simulink model "SIMQGC"  (R2017a)
settings: Solver=VariableStepAuto  StartTime=0.0  StopTime=1000  RelTol=1e-3
model workspace: external: MAT-File (data not in the file)
values from neighbouring files (symbols this model uses):
  aDe =     [MY3.mat]
  aDyn =     [MY3.mat]
  aLat =     [MY3.mat]
  aLon =     [MY3.mat]
  H = HGround + geo.Zgear + GearData.R - MCdata.mass*9.8/4/GearData.Sp    [my3_acdata.m]
  HGround = 500    [my3_acdata.m]
  phi_max = 20    [my3_acdata.m]
  phi_min = -20    [my3_acdata.m]
  psi_max = 30    [my3_acdata.m]
  psi_min = -30    [my3_acdata.m]
  theta_max = 20    [my3_acdata.m]
  theta_min = -20    [my3_acdata.m]
  Xmax = 0.01    [my3_acdata.m]
  Xmin = 0    [my3_acdata.m]
  Ymax = 0.01    [my3_acdata.m]
  Ymin = 0    [my3_acdata.m]
  Zmax = 0.01    [my3_acdata.m]
  Zmin = 0    [my3_acdata.m]
undefined symbols (not defined in the file or in its folder): Earth, geo, ini, magnitude, Motor, Newton, Prop, Raphson, Standard_Devices, UDP_Protocol, WGS84
undefined symbols (not defined in the file): GearData, LProp, RProp
libraries: simulink_extras x12, dspnetwork x8, aerolibobsolete x6, sharedutil x6, simulink x4, aerolibfltsims x3, aerolibasang x2, aerolibatmos2 x1, aerolibbdyn x1, aerolibtransform2 x1, aerolibanimutils x1, sldrtlib x1
(part 2 of 3)

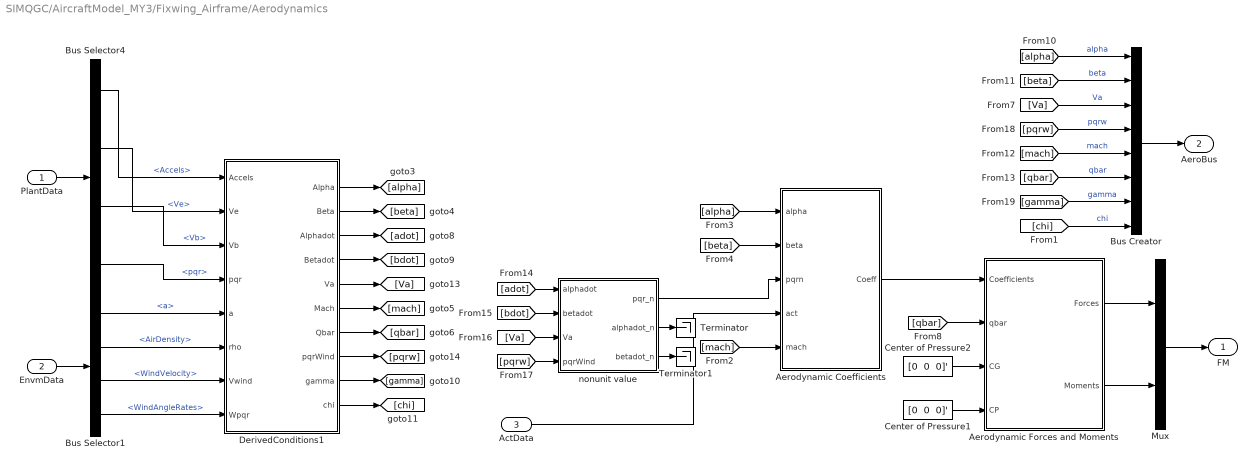
== system SIMQGC/AircraftModel_MY3/Fixwing_Airframe/Aerodynamics ==
  PlantData : Inport
  EnvmData : Inport  Port=2
  ActData : Inport  Port=3
  Aerodynamic Coefficients : Subsystem  AncestorBlock=asbhl20vehicle/Vehicle/Aerodynamic/Aerodynamic Coefficients
  Aerodynamic Forces and Moments : Subsystem  mask(Aerodynamic Forces and Moments){S=geo.Sw, b=geo.b, cbar=geo.MAC}
      mask prompts: S "Reference area:"; b "Reference span:"; cbar "Reference length:"
      mask help: Compute the aerodynamic forces and moments applied at the center of gravity using the aerodynamic coefficients, dynamic pressure, center of gravity and center of pressure.
      mask Help: web(asbhelp);
      mask Display:
      | port_label('input',1,'Coefficients','texmode','on');
      | port_label('input',2,'q_{bar}','texmode','on');
      | port_label('input',3,'CG','texmode','on');
      | port_label('input',4,'CP','texmode','on');
      | port_label('output',1,'F_{aero}','texmode','on');
      | port_label('output',2,'M_{aero}','texmode','on');
  Bus Creator : BusCreator  Inputs=8
  Bus Selector1 : BusSelector  OutputSignals=a,AirDensity,WindVelocity,WindAngleRates
  Bus Selector4 : BusSelector  OutputSignals=Accels,Ve,Vb,pqr
  Center of Pressure1 : Constant  Value="[0  0  0]'"  SampleTime=0
  Center of Pressure2 : Constant  Value="[0  0  0]'"  SampleTime=0
  DerivedConditions1 : Subsystem
  Mux : Mux  Inputs=2
  Terminator : Terminator
  Terminator1 : Terminator
  nonunit value : Subsystem
  FM : Outport  PortDimensions=6
  AeroBus : Outport  Port=2
  wires:
  Aerodynamic Forces and Moments/1(Forces) -> Mux/1
  PlantData/1 -> Bus Selector4/1
  EnvmData/1 -> Bus Selector1/1
  Bus Creator/1 -> AeroBus/1
  [qbar] -> Aerodynamic Forces and Moments/2(qbar)
  Bus Selector4/1 -> DerivedConditions1/1(Accels)  "<Accels>"
  Bus Selector4/2 -> DerivedConditions1/2(Ve)  "<Ve>"
  Bus Selector4/3 -> DerivedConditions1/3(Vb)  "<Vb>"
  Bus Selector4/4 -> DerivedConditions1/4(pqr)  "<pqr>"
  Bus Selector1/1 -> DerivedConditions1/5(a)  "<a>"
  Bus Selector1/2 -> DerivedConditions1/6(rho)  "<AirDensity>"
  Bus Selector1/3 -> DerivedConditions1/7(Vwind)  "<WindVelocity>"
  Bus Selector1/4 -> DerivedConditions1/8(Wpqr)  "<WindAngleRates>"
  DerivedConditions1/1(Alpha) -> [alpha]
  DerivedConditions1/2(Beta) -> [beta]
  DerivedConditions1/5(Va) -> [Va]
  DerivedConditions1/6(Mach) -> [mach]
  DerivedConditions1/7(Qbar) -> [qbar]
  DerivedConditions1/8(pqrWind) -> [pqrw]
  DerivedConditions1/9(gamma) -> [gamma]
  DerivedConditions1/10(chi) -> [chi]
  [alpha] -> Bus Creator/1  "alpha"
  [beta] -> Bus Creator/2  "beta"
  [Va] -> Bus Creator/3  "Va"
  [pqrw] -> Bus Creator/4  "pqrw"
  [mach] -> Bus Creator/5  "mach"
  [qbar] -> Bus Creator/6  "qbar"
  [gamma] -> Bus Creator/7  "gamma"
  Aerodynamic Forces and Moments/2(Moments) -> Mux/2
  Mux/1 -> FM/1
  DerivedConditions1/3(Alphadot) -> [adot]
  DerivedConditions1/4(Betadot) -> [bdot]
  [adot] -> nonunit value/1(alphadot)
  [bdot] -> nonunit value/2(betadot)
  [Va] -> nonunit value/3(Va)
  [pqrw] -> nonunit value/4(pqrWind)
  [alpha] -> Aerodynamic Coefficients/1(alpha)
  [beta] -> Aerodynamic Coefficients/2(beta)
  nonunit value/1(pqr_n) -> Aerodynamic Coefficients/3(pqrn)
  nonunit value/2(alphadot_n) -> Terminator/1
  nonunit value/3(betadot_n) -> Terminator1/1
  Center of Pressure2/1 -> Aerodynamic Forces and Moments/3(CG)
  Center of Pressure1/1 -> Aerodynamic Forces and Moments/4(CP)
  ActData/1 -> Aerodynamic Coefficients/4(act)
  [chi] -> Bus Creator/8  "chi"
  [mach] -> Aerodynamic Coefficients/5(mach)
  Aerodynamic Coefficients/1(Coeff) -> Aerodynamic Forces and Moments/1(Coefficients)

== system SIMQGC/AircraftModel_MY3/Fixwing_Airframe/Gravity ==
  PlantData : Inport
  Bus Selector1 : BusSelector  OutputSignals=gb
  Constant1 : Constant  Value=ini.mass
  Constant3 : Constant  Value=[0 0 0]'
  Constant4 : Constant  Value=geo.Xcg
  Constant5 : Constant  Value=0
  Constant6 : Constant  Value=0
  Mux1 : Mux  Inputs=2
  Mux2 : Mux  Inputs=3
  Product : Product  RndMeth=Zero
  FM : Outport  PortDimensions=6
  mass : Outport  Port=2
  CG : Outport  Port=3
  wires:
  PlantData/1 -> Bus Selector1/1
  Constant3/1 -> Mux1/2
  Mux1/1 -> FM/1
  Bus Selector1/1 -> Product/1  "<gb>"
  Product/1 -> Mux1/1
  Constant1/1 -> Product/2, mass/1
  Mux2/1 -> CG/1
  Constant4/1 -> Mux2/1
  Constant5/1 -> Mux2/2
  Constant6/1 -> Mux2/3

== system SIMQGC/AircraftModel_MY3/Fixwing_Airframe/GroundForces ==
  PlantData : Inport
  Bus Creator : BusCreator  Inputs=4
  Constant : Constant  Value=HGround
  LF_Gear : Subsystem  AncestorBlock=|  TreatAsAtomicUnit=on  mask(simple aircraft undercarriage){loc=GearData.PLF, Rw=GearData.R, Ks=GearData.Sp, Cs=GearData.Damp, Rcs=GearData.CompMax, muroll=GearData.muRoll, A=GearData.muA, B=GearData.muB}
      | asbhl20vehicle/Vehicle/LandingGear
      | GroundReaction/L Main Gear Geometry
      | Forces and Moments
      mask prompts: loc "Gear location"; Rw "Wheel radius"; Ks "Strut Spring rate"; Cs "Strut Damping rate"; Rcs "Strut compress range"; muroll "Tire roll friction coefficient"; A "Tire friction caculate experience formula parameter A"; B "Tire friction caculate experience formula parameter B"
      mask help:
      | the model descripes the basic mechanics model according to  geoometry
      | relationship. there are no brake device model, and no hydraulic model etc,
      | only the basic forces and moments caculation in the model.
      | it is designed to be appllied to small uav.
  LM_Gear : Subsystem  AncestorBlock=|  TreatAsAtomicUnit=on  mask(simple aircraft undercarriage){loc=GearData.PLM, Rw=GearData.R, Ks=GearData.Sp, Cs=GearData.Damp, Rcs=GearData.CompMax, muroll=GearData.muRoll, A=GearData.muA, B=GearData.muB}
      | asbhl20vehicle/Vehicle/LandingGear
      | GroundReaction/L Main Gear Geometry
      | Forces and Moments
      mask prompts: loc "Gear location"; Rw "Wheel radius"; Ks "Strut Spring rate"; Cs "Strut Damping rate"; Rcs "Strut compress range"; muroll "Tire roll friction coefficient"; A "Tire friction caculate experience formula parameter A"; B "Tire friction caculate experience formula parameter B"
      mask help:
      | the model descripes the basic mechanics model according to  geoometry
      | relationship. there are no brake device model, and no hydraulic model etc,
      | only the basic forces and moments caculation in the model.
      | it is designed to be appllied to small uav.
  LN_Gear : Subsystem  AncestorBlock=|  TreatAsAtomicUnit=on  mask(simple aircraft undercarriage){loc=GearData.PRM, Rw=GearData.R, Ks=GearData.Sp, Cs=GearData.Damp, Rcs=GearData.CompMax, muroll=GearData.muRoll, A=GearData.muA, B=GearData.muB}
      | asbhl20vehicle/Vehicle/LandingGear
      | GroundReaction/L Main Gear Geometry
      | Forces and Moments
      mask prompts: loc "Gear location"; Rw "Wheel radius"; Ks "Strut Spring rate"; Cs "Strut Damping rate"; Rcs "Strut compress range"; muroll "Tire roll friction coefficient"; A "Tire friction caculate experience formula parameter A"; B "Tire friction caculate experience formula parameter B"
      mask help:
      | the model descripes the basic mechanics model according to  geoometry
      | relationship. there are no brake device model, and no hydraulic model etc,
      | only the basic forces and moments caculation in the model.
      | it is designed to be appllied to small uav.
  RF_Gear : Subsystem  AncestorBlock=|  TreatAsAtomicUnit=on  mask(simple aircraft undercarriage){loc=GearData.PRF, Rw=GearData.R, Ks=GearData.Sp, Cs=GearData.Damp, Rcs=GearData.CompMax, muroll=GearData.muRoll, A=GearData.muA, B=GearData.muB}
      | asbhl20vehicle/Vehicle/LandingGear
      | GroundReaction/L Main Gear Geometry
      | Forces and Moments
      mask prompts: loc "Gear location"; Rw "Wheel radius"; Ks "Strut Spring rate"; Cs "Strut Damping rate"; Rcs "Strut compress range"; muroll "Tire roll friction coefficient"; A "Tire friction caculate experience formula parameter A"; B "Tire friction caculate experience formula parameter B"
      mask help:
      | the model descripes the basic mechanics model according to  geoometry
      | relationship. there are no brake device model, and no hydraulic model etc,
      | only the basic forces and moments caculation in the model.
      | it is designed to be appllied to small uav.
  Sum : Sum  Inputs=++++
  Terminator{,1..3} (4 alike) : Terminator
  FM : Outport
  WOW : Outport  Port=2
  wires:
  PlantData/1 -> RF_Gear/1(PlantData), LN_Gear/1(PlantData), LM_Gear/1(PlantData), LF_Gear/1(PlantData)
  Constant/1 -> RF_Gear/2(runway height), LN_Gear/2(runway height), LM_Gear/2(runway height), LF_Gear/2(runway height)
  LF_Gear/3(FM) -> Sum/1
  RF_Gear/3(FM) -> Sum/2
  LM_Gear/3(FM) -> Sum/3
  LN_Gear/3(FM) -> Sum/4
  Sum/1 -> FM/1
  LF_Gear/1(WOW) -> [LF]
  RF_Gear/1(WOW) -> [RF]
  LM_Gear/1(WOW) -> [LM]
  LN_Gear/1(WOW) -> [RM]
  [RF] -> Bus Creator/2  "RF"
  Bus Creator/1 -> WOW/1
  [LF] -> Bus Creator/1  "LF"
  [LM] -> Bus Creator/3  "LM"
  [RM] -> Bus Creator/4  "RM"
  LF_Gear/2(S) -> Terminator/1
  RF_Gear/2(S) -> Terminator1/1
  LM_Gear/2(S) -> Terminator2/1
  LN_Gear/2(S) -> Terminator3/1

== system SIMQGC/AircraftModel_MY3/Fixwing_Airframe/PlantBus ==
  Ve : Inport
  Xe : Inport  Port=2
  Euler : Inport  Port=3
  DCM : Inport  Port=4
  Vb : Inport  Port=5
  pqr : Inport  Port=6
  pqrdot : Inport  Port=7
  Accels : Inport  Port=8
  AeroBus : Inport  Port=9
  EnvmData : Inport  Port=10
  mass : Inport  Port=11
  CG : Inport  Port=12
  ACTData : Inport  Port=13
  WOW : Inport  Port=14
  5 : Selector  InputPortWidth=3  IndexOptions=Index vector (dialog)  Indices=3  OutputSizes=1
  Bus Selector1 : BusSelector  OutputSignals=alpha,beta,Va,pqrw,mach,qbar,gamma,chi
  Bus Selector4 : BusSelector  OutputSignals=hground,g,To,Po
  Gain : Gain  Gain=-1
  PlantBus : BusCreator  Inputs=26
  Subsystem : Subsystem
  Sum : Sum  Inputs=+-|
  "nb & gb " : Subsystem
  Data : Outport
  wires:
  Euler/1 -> Subsystem/1(Ein)
  PlantBus/1 -> Data/1  "PlantBus"
  AeroBus/1 -> Bus Selector1/1
  EnvmData/1 -> Bus Selector4/1
  Ve/1 -> PlantBus/1  "Ve"
  Xe/1 -> PlantBus/2, 5/1  "Xe"
  5/1 -> Gain/1
  Gain/1 -> PlantBus/3, Sum/1  "H"
  DCM/1 -> PlantBus/6, "nb & gb "/1(DCM)  "DCM"
  Bus Selector4/1 -> Sum/2  "<hground>"
  Accels/1 -> PlantBus/20, "nb & gb "/3(a)  "Accels"
  Bus Selector4/2 -> "nb & gb "/2(g)  "<g>"
  Sum/1 -> PlantBus/4  "Hag"
  Subsystem/1(E) -> PlantBus/5  "Euler"
  Vb/1 -> PlantBus/7  "Vb"
  pqr/1 -> PlantBus/8  "pqr"
  pqrdot/1 -> PlantBus/9  "pqrdot"
  "nb & gb "/1(nb) -> PlantBus/10  "nb"
  "nb & gb "/2(gb) -> PlantBus/11  "gb"
  Bus Selector1/1 -> PlantBus/12  "<alpha>"
  Bus Selector1/2 -> PlantBus/13  "<beta>"
  Bus Selector1/3 -> PlantBus/14  "<Va>"
  Bus Selector1/4 -> PlantBus/15  "<pqrw>"
  Bus Selector1/5 -> PlantBus/16  "<mach>"
  Bus Selector1/6 -> PlantBus/17  "<qbar>"
  Bus Selector1/7 -> PlantBus/18  "<gamma>"
  Bus Selector1/8 -> PlantBus/19  "<chi>"
  mass/1 -> PlantBus/21  "mass"
  CG/1 -> PlantBus/22  "CG"
  ACTData/1 -> PlantBus/23  "ACTData"
  WOW/1 -> PlantBus/24  "WOW"
  Bus Selector4/3 -> PlantBus/25  "<To>"
  Bus Selector4/4 -> PlantBus/26  "<Po>"

== system SIMQGC/AircraftModel_MY3/Fixwing_Airframe/Propulsion ==
  ActData : Inport
  PlantData : Inport  Port=2
  EnvData : Inport  Port=3
  ActData1 : InportShadow
  Bus Selector : BusSelector  OutputSignals=dtl
  Bus Selector1 : BusSelector  OutputSignals=Va
  Bus Selector2 : BusSelector  OutputSignals=AirDensity
  Bus Selector3 : BusSelector  OutputSignals=dtr
  Bus Selector4 : BusSelector  OutputSignals=pqr
  Gain : Gain  Gain=Prop.Y
  Left_MotorAndPropeller : Subsystem  mask{P=LProp.P, C=LProp.C}
      mask prompts: P "Assemble Position in Body Frame(m)"; C "Spin Direction(-1 for clockwise,1 for countted clockwise)"
      mask DialogControl DescTextVar Prompt: Motor and Propeller Model
  Right_MotorAndPropeller : Subsystem  mask{P=RProp.P, C=RProp.C}
      mask prompts: P "Assemble Position in Body Frame(m)"; C "Spin Direction(-1 for clockwise,1 for countted clockwise)"
      mask DialogControl DescTextVar Prompt: Motor and Propeller Model
  Selector : Selector  InputPortWidth=3  IndexOptions=Index vector (dialog)  Indices=[3]  OutputSizes=1
  Sum : Sum  Inputs=|++
  Sum1 : Sum  Inputs=|++
  Sum2 : Sum  Inputs=+-|
  FM : Outport  PortDimensions=6  InitialOutput=0
  wires:
  ActData/1 -> Bus Selector/1
  PlantData/1 -> Bus Selector4/1, Bus Selector1/1
  Bus Selector/1 -> Left_MotorAndPropeller/1(dt)  "<dtl>"
  Bus Selector1/1 -> Sum2/1, Sum1/1  "<Va>"
  EnvData/1 -> Bus Selector2/1
  Bus Selector2/1 -> Right_MotorAndPropeller/3(rho), Left_MotorAndPropeller/3(rho)  "<AirDensity>"
  ActData1/1 -> Bus Selector3/1
  Bus Selector3/1 -> Right_MotorAndPropeller/1(dt)  "<dtr>"
  Left_MotorAndPropeller/1(FM) -> Sum/1
  Right_MotorAndPropeller/1(FM) -> Sum/2
  Sum/1 -> FM/1
  Sum1/1 -> Left_MotorAndPropeller/2(V)
  Bus Selector4/1 -> Selector/1  "<pqr>"
  Selector/1 -> Gain/1
  Gain/1 -> Sum2/2, Sum1/2
  Sum2/1 -> Right_MotorAndPropeller/2(V)

== system SIMQGC/UDPReadFromQGC/Subsystem/joystick ==
  data : Inport
  Action Port : ActionPort  ActionType=case
  Demux : Demux  Outputs=8
  Mux : Mux  Inputs=3
  Terminator{,1..4} (5 alike) : Terminator
  joystick : Outport
  wires:
  data/1 -> Demux/1
  Demux/1 -> Mux/1
  Demux/2 -> Mux/2
  Demux/3 -> Mux/3
  Mux/1 -> joystick/1
  Demux/4 -> Terminator/1
  Demux/5 -> Terminator1/1
  Demux/6 -> Terminator2/1
  Demux/7 -> Terminator3/1
  Demux/8 -> Terminator4/1

== system SIMQGC/UDPReadFromQGC/Subsystem/throttle ==
  data : Inport
  Action Port : ActionPort  ActionType=case
  Demux : Demux  Outputs=8
  Mux : Mux  Inputs=2
  Terminator{,1..5} (6 alike) : Terminator
  throttle : Outport
  wires:
  data/1 -> Demux/1
  Demux/1 -> Mux/1
  Demux/2 -> Mux/2
  Demux/3 -> Terminator5/1
  Mux/1 -> throttle/1
  Demux/4 -> Terminator/1
  Demux/5 -> Terminator1/1
  Demux/6 -> Terminator2/1
  Demux/7 -> Terminator3/1
  Demux/8 -> Terminator4/1

== system SIMQGC/AircraftModel_MY3/Fixwing_Airframe/Aerodynamics/Aerodynamic Coefficients ==
  alpha : Inport
  beta : Inport  Port=2
  pqrn : Inport  Port=3
  act : Inport  Port=4
  mach : Inport  Port=5
  Basic Coefficients : Subsystem
  Body Rate Damping : Subsystem
  LY0 : Gain
  LY1 : Gain
  Mux1 : Mux  Inputs=2
  Selector : Selector  InputPortWidth=6  IndexOptions=Index vector (dialog)  Indices=[1 2 3]  OutputSizes=1
  Selector1 : Selector  InputPortWidth=6  IndexOptions=Index vector (dialog)  Indices=[4 5 6]  OutputSizes=1
  Sum : Sum  Inputs=3  SaturateOnIntegerOverflow=on  InputSameDT=on  OutDataTypeStr=Inherit: Same as first input
  actuator : Subsystem
  body axis forces : Subsystem
  Coeff : Outport  InitialOutput=0
  wires:
  alpha/1 -> body axis forces/1(alpha), Body Rate Damping/1(alpha), actuator/1(alpha), Basic Coefficients/1(alpha)
  beta/1 -> body axis forces/2(beta), Basic Coefficients/2(beta)
  pqrn/1 -> Body Rate Damping/2(pqrn)
  Body Rate Damping/1(coeff) -> Sum/2
  Basic Coefficients/1(coeff) -> Sum/1
  actuator/1(coeff) -> Sum/3
  act/1 -> actuator/2(act)
  mach/1 -> Basic Coefficients/3(mach)
  Selector1/1 -> LY1/1
  Mux1/1 -> Coeff/1
  Selector/1 -> LY0/1
  Sum/1 -> Selector1/1, Selector/1
  body axis forces/1(Cl_XYZ) -> Mux1/1
  LY0/1 -> body axis forces/3(Cl_LDY)
  LY1/1 -> Mux1/2

== system SIMQGC/AircraftModel_MY3/Fixwing_Airframe/Aerodynamics/Aerodynamic Forces and Moments ==
  Coefficients : Inport
  qbar : Inport  Port=2
  CG : Inport  Port=3
  CP : Inport  Port=4
  Demux1 : Demux  Outputs=[3,3]
  Moments about CG due to Forces : aerolibbdyn/Moments about CG  due to Forces
      settings: SourceProductName=Aerospace Blockset  SourceProductBaseCode=AE
  Product : Product  SaturateOnIntegerOverflow=on  InputSameDT=on  OutDataTypeStr=Inherit: Same as first input
  Product3 : Product  SaturateOnIntegerOverflow=on  InputSameDT=on  OutDataTypeStr=Inherit: Same as first input
  Sum1 : Sum  Inputs=++|  SaturateOnIntegerOverflow=on  InputSameDT=on  OutDataTypeStr=Inherit: Same as first input
  reference area : Gain  Gain=S  SaturateOnIntegerOverflow=on  OutDataTypeStr=Inherit: Same as input  ParamDataTypeStr=Inherit: Same as input
  reference length : Gain  Gain=[b cbar b]  SaturateOnIntegerOverflow=on  OutDataTypeStr=Inherit: Same as input  ParamDataTypeStr=Inherit: Same as input
  Forces : Outport
  Moments : Outport  Port=2
  wires:
  Moments about CG due to Forces/1 -> Sum1/1
  reference length/1 -> Product3/2
  Coefficients/1 -> Demux1/1
  Demux1/1 -> Product/2
  Demux1/2 -> Product3/1
  qbar/1 -> reference area/1
  reference area/1 -> reference length/1, Product/1
  Product/1 -> Forces/1, Moments about CG due to Forces/1
  Product3/1 -> Sum1/2
  Sum1/1 -> Moments/1
  CG/1 -> Moments about CG due to Forces/2
  CP/1 -> Moments about CG due to Forces/3

== system SIMQGC/AircraftModel_MY3/Fixwing_Airframe/Aerodynamics/DerivedConditions1 ==
  Accels : Inport
  Ve : Inport  Port=2
  Vb : Inport  Port=3
  pqr : Inport  Port=4
  a : Inport  Port=5
  rho : Inport  Port=6
  Vwind : Inport  Port=7
  Wpqr : Inport  Port=8
  Derivative : Derivative
  Derivative1 : Derivative
  Dynamic Pressure : aerolibasang/Dynamic Pressure
  "Incidence, Sideslip, & Airspeed" : Subsystem  AncestorBlock=aerolibasang/Incidence, Sideslip, & Airspeed  mask(Incidence,Sideslip,&Airspeed){}
      mask help: aeroblks:aeroblkasang:blockIncidenceSideslipAirspeedDesc
      mask init:
      | aeroicon('aeroblk');
      mask Help: eval('asbhelp(''incidence_sideslip_and_airspeed'')');
      mask Display:
      | port_label('input',1,'V_b','texmode','on');
      | port_label('output',1,'\alpha','texmode','on');
      | port_label('output',2,'\beta','texmode','on');
      | port_label('output',3,'V','texmode','on');
  Mach Number : aerolibasang/Mach Number
      settings: SourceProductName=Aerospace Blockset  SourceProductBaseCode=AE
  Saturation1 : Saturate  UpperLimit=40/57.3  LowerLimit=-40/57.3
  Sum1 : Sum  Inputs=++|  SaturateOnIntegerOverflow=on  InputSameDT=on  OutDataTypeStr=Inherit: Same as first input
  Sum2 : Sum  Inputs=|+-  SaturateOnIntegerOverflow=on  InputSameDT=on  OutDataTypeStr=Inherit: Same as first input
  Terminator : Terminator
  Terminator1 : Terminator
  Terminator2 : Terminator
  gamma chi & speed : Subsystem  AncestorBlock=cldesignlib/Aircraft Dynamics/gamma chi & speed  mask(flight path angle & speed){}
      mask help: Calculate the angles between the velocity vector and the ground under NED coordinate (Ve).
      mask Display:
      | port_label('input',1,'V_e','texmode','on');
      | port_label('output',1,'\gamma','texmode','on');
      | port_label('output',2,'\chi','texmode','on');
      | port_label('output',3,'V','texmode','on');
  pqr1 : InportShadow  Port=4
  Alpha : Outport
  Beta : Outport  Port=2
  Alphadot : Outport  Port=3
  Betadot : Outport  Port=4
  Va : Outport  Port=5
  Mach : Outport  Port=6
  Qbar : Outport  Port=7
  pqrWind : Outport  Port=8
  gamma : Outport  Port=9
  chi : Outport  Port=10
  wires:
  gamma chi & speed/2(chi) -> chi/1
  gamma chi & speed/1(gamma) -> gamma/1
  Ve/1 -> gamma chi & speed/1(Ve)
  Vwind/1 -> Sum2/2
  "Incidence, Sideslip, & Airspeed"/1(Alpha) -> Alpha/1, Derivative/1
  Sum1/1 -> pqrWind/1
  pqr/1 -> Sum1/1
  Wpqr/1 -> Sum1/2
  rho/1 -> Dynamic Pressure/2
  a/1 -> Mach Number/2
  Vb/1 -> Sum2/1
  Mach Number/1 -> Mach/1
  "Incidence, Sideslip, & Airspeed"/3(V) -> Va/1
  "Incidence, Sideslip, & Airspeed"/2(Beta) -> Saturation1/1
  Sum2/1 -> "Incidence, Sideslip, & Airspeed"/1(Vb), Dynamic Pressure/1, Mach Number/1
  Saturation1/1 -> Beta/1, Derivative1/1
  Derivative/1 -> Alphadot/1
  Derivative1/1 -> Betadot/1
  Dynamic Pressure/1 -> Qbar/1
  gamma chi & speed/3(V) -> Terminator2/1
  pqr1/1 -> Terminator/1
  Accels/1 -> Terminator1/1

== system SIMQGC/AircraftModel_MY3/Fixwing_Airframe/Aerodynamics/nonunit value ==
  alphadot : Inport
  betadot : Inport  Port=2
  Va : Inport  Port=3
  pqrWind : Inport  Port=4
  Demux2 : Demux  Outputs=3
  Gain : Gain  Gain=2  SaturateOnIntegerOverflow=on  OutDataTypeStr=Inherit: Same as input  ParamDataTypeStr=Inherit: Same as input
  Mux18 : Mux  Inputs=3
  Product{1..5} (5 alike) : Product  Inputs=/**  SaturateOnIntegerOverflow=on  OutDataTypeStr=Inherit: Same as first input
  Saturation : Saturate  UpperLimit=inf  LowerLimit=0.1
  b : Constant  Value=geo.b
  c : Constant  Value=geo.MAC
  pqr_n : Outport
  alphadot_n : Outport  Port=2
  betadot_n : Outport  Port=3
  wires:
  alphadot/1 -> Product3/3
  Product3/1 -> alphadot_n/1
  Saturation/1 -> Product2/1, Product3/1, Product5/1, Product4/1, Product1/1
  Product1/1 -> Mux18/1
  Mux18/1 -> pqr_n/1
  c/1 -> Product3/2, Product4/2
  Demux2/1 -> Product1/3
  Demux2/2 -> Product4/3
  Demux2/3 -> Product2/3
  b/1 -> Product1/2, Product2/2, Product5/2
  Gain/1 -> Saturation/1
  Product2/1 -> Mux18/3
  Product4/1 -> Mux18/2
  Va/1 -> Gain/1
  pqrWind/1 -> Demux2/1
  betadot/1 -> Product5/3
  Product5/1 -> betadot_n/1

== system SIMQGC/AircraftModel_MY3/Fixwing_Airframe/GroundForces/LF_Gear ==
  PlantData : Inport
  runway height : Inport  Port=2
  Bus Selector1 : BusSelector  OutputSignals=DCM,Xe,Vb,pqr,Euler
  Gain2 : Gain  Gain=-1
  GenerateGroundFM1 : Subsystem  TreatAsAtomicUnit=on
  detect ground contact : Subsystem
  gear location : Constant  Value=loc
  psi : Selector  InputPortWidth=3  IndexOptions=Index vector (dialog)  Indices=3  OutputSizes=1
  ze : Selector  InputPortWidth=3  IndexOptions=Index vector (dialog)  Indices=3  OutputSizes=1
  WOW : Outport
  S : Outport  Port=2
  FM : Outport  Port=3
  wires:
  GenerateGroundFM1/1(S) -> S/1
  Gain2/1 -> GenerateGroundFM1/1(zrw)
  gear location/1 -> GenerateGroundFM1/2(Xgb), detect ground contact/3(Xgb)
  psi/1 -> GenerateGroundFM1/7(psi)
  Bus Selector1/4 -> GenerateGroundFM1/6(pqr)  "<pqr>"
  Bus Selector1/3 -> GenerateGroundFM1/5(Vb)  "<Vb>"
  Bus Selector1/1 -> GenerateGroundFM1/3(DCM), detect ground contact/2(DCM)  "<DCM>"
  ze/1 -> GenerateGroundFM1/4(ze), detect ground contact/1(ze)
  Bus Selector1/2 -> ze/1  "<Xe>"
  runway height/1 -> Gain2/1, detect ground contact/4(Hrw)
  Bus Selector1/5 -> psi/1  "<Euler>"
  GenerateGroundFM1/2(FM) -> FM/1
  PlantData/1 -> Bus Selector1/1
  detect ground contact/1(WOW) -> GenerateGroundFM1/Enable, WOW/1

== system SIMQGC/AircraftModel_MY3/Fixwing_Airframe/GroundForces/LM_Gear ==
  note: Left main gear
  PlantData : Inport
  runway height : Inport  Port=2
  Bus Selector1 : BusSelector  OutputSignals=DCM,Xe,Vb,pqr,Euler
  Gain2 : Gain  Gain=-1
  GenerateGroundFM1 : Subsystem  TreatAsAtomicUnit=on
  detect ground contact : Subsystem
  gear location : Constant  Value=loc
  psi : Selector  InputPortWidth=3  IndexOptions=Index vector (dialog)  Indices=3  OutputSizes=1
  ze : Selector  InputPortWidth=3  IndexOptions=Index vector (dialog)  Indices=3  OutputSizes=1
  WOW : Outport
  S : Outport  Port=2
  FM : Outport  Port=3
  wires:
  GenerateGroundFM1/1(S) -> S/1
  Gain2/1 -> GenerateGroundFM1/1(zrw)
  gear location/1 -> GenerateGroundFM1/2(Xgb), detect ground contact/3(Xgb)
  psi/1 -> GenerateGroundFM1/7(psi)
  Bus Selector1/4 -> GenerateGroundFM1/6(pqr)  "<pqr>"
  Bus Selector1/3 -> GenerateGroundFM1/5(Vb)  "<Vb>"
  Bus Selector1/1 -> GenerateGroundFM1/3(DCM), detect ground contact/2(DCM)  "<DCM>"
  ze/1 -> GenerateGroundFM1/4(ze), detect ground contact/1(ze)
  Bus Selector1/2 -> ze/1  "<Xe>"
  runway height/1 -> Gain2/1, detect ground contact/4(Hrw)
  Bus Selector1/5 -> psi/1  "<Euler>"
  GenerateGroundFM1/2(FM) -> FM/1
  PlantData/1 -> Bus Selector1/1
  detect ground contact/1(WOW) -> GenerateGroundFM1/Enable, WOW/1

== system SIMQGC/AircraftModel_MY3/Fixwing_Airframe/GroundForces/LN_Gear ==
  note: Left main gear
  PlantData : Inport
  runway height : Inport  Port=2
  Bus Selector1 : BusSelector  OutputSignals=DCM,Xe,Vb,pqr,Euler
  Gain2 : Gain  Gain=-1
  GenerateGroundFM1 : Subsystem  TreatAsAtomicUnit=on
  detect ground contact : Subsystem
  gear location : Constant  Value=loc
  psi : Selector  InputPortWidth=3  IndexOptions=Index vector (dialog)  Indices=3  OutputSizes=1
  ze : Selector  InputPortWidth=3  IndexOptions=Index vector (dialog)  Indices=3  OutputSizes=1
  WOW : Outport
  S : Outport  Port=2
  FM : Outport  Port=3
  wires:
  PlantData/1 -> Bus Selector1/1
  GenerateGroundFM1/2(FM) -> FM/1
  Bus Selector1/5 -> psi/1  "<Euler>"
  runway height/1 -> detect ground contact/4(Hrw), Gain2/1
  Bus Selector1/2 -> ze/1  "<Xe>"
  ze/1 -> GenerateGroundFM1/4(ze), detect ground contact/1(ze)
  Bus Selector1/1 -> GenerateGroundFM1/3(DCM), detect ground contact/2(DCM)  "<DCM>"
  Bus Selector1/3 -> GenerateGroundFM1/5(Vb)  "<Vb>"
  Bus Selector1/4 -> GenerateGroundFM1/6(pqr)  "<pqr>"
  psi/1 -> GenerateGroundFM1/7(psi)
  gear location/1 -> GenerateGroundFM1/2(Xgb), detect ground contact/3(Xgb)
  Gain2/1 -> GenerateGroundFM1/1(zrw)
  GenerateGroundFM1/1(S) -> S/1
  detect ground contact/1(WOW) -> GenerateGroundFM1/Enable, WOW/1

== system SIMQGC/AircraftModel_MY3/Fixwing_Airframe/GroundForces/RF_Gear ==
  note: Left main gear
  PlantData : Inport
  runway height : Inport  Port=2
  Bus Selector1 : BusSelector  OutputSignals=DCM,Xe,Vb,pqr,Euler
  Gain2 : Gain  Gain=-1
  GenerateGroundFM1 : Subsystem  TreatAsAtomicUnit=on
  detect ground contact : Subsystem
  gear location : Constant  Value=loc
  psi : Selector  InputPortWidth=3  IndexOptions=Index vector (dialog)  Indices=3  OutputSizes=1
  ze : Selector  InputPortWidth=3  IndexOptions=Index vector (dialog)  Indices=3  OutputSizes=1
  WOW : Outport
  S : Outport  Port=2
  FM : Outport  Port=3
  wires:
  PlantData/1 -> Bus Selector1/1
  GenerateGroundFM1/2(FM) -> FM/1
  Bus Selector1/5 -> psi/1  "<Euler>"
  runway height/1 -> detect ground contact/4(Hrw), Gain2/1
  Bus Selector1/2 -> ze/1  "<Xe>"
  ze/1 -> GenerateGroundFM1/4(ze), detect ground contact/1(ze)
  Bus Selector1/1 -> GenerateGroundFM1/3(DCM), detect ground contact/2(DCM)  "<DCM>"
  Bus Selector1/3 -> GenerateGroundFM1/5(Vb)  "<Vb>"
  Bus Selector1/4 -> GenerateGroundFM1/6(pqr)  "<pqr>"
  psi/1 -> GenerateGroundFM1/7(psi)
  gear location/1 -> GenerateGroundFM1/2(Xgb), detect ground contact/3(Xgb)
  Gain2/1 -> GenerateGroundFM1/1(zrw)
  GenerateGroundFM1/1(S) -> S/1
  detect ground contact/1(WOW) -> GenerateGroundFM1/Enable, WOW/1

== system SIMQGC/AircraftModel_MY3/Fixwing_Airframe/PlantBus/Subsystem ==
  note: trasfer psi to [-pi pi]
  Ein : Inport
  Constant1 : Constant  Value=2*pi
  Constant3 : Constant  Value=pi
  Demux : Demux  Outputs=3
  Math Function : Math  Operator=mod  SaturateOnIntegerOverflow=on
  Subtract : Sum  Inputs=+-
  Subtract1 : Sum
  Vector Concatenate : Concatenate  NumInputs=3
  E : Outport
  wires:
  Constant1/1 -> Math Function/2
  Math Function/1 -> Subtract/1
  Subtract1/1 -> Math Function/1
  Constant3/1 -> Subtract1/2, Subtract/2
  Demux/3 -> Subtract1/1
  Subtract/1 -> Vector Concatenate/3
  Ein/1 -> Demux/1
  Demux/1 -> Vector Concatenate/1
  Demux/2 -> Vector Concatenate/2
  Vector Concatenate/1 -> E/1

== system SIMQGC/AircraftModel_MY3/Fixwing_Airframe/PlantBus/nb & gb  ==
  DCM : Inport
  g : Inport  Port=2
  a : Inport  Port=3
  Constant : Constant  Value=[1 1 -1]
  Divide : Product  Inputs=*/
  Product : Product  RndMeth=Zero
  Sum2 : Sum  Inputs=|+-
  cal gb : Subsystem
  nb : Outport
  gb : Outport  Port=2
  wires:
  Product/1 -> nb/1
  Constant/1 -> Product/2
  Divide/1 -> Product/1
  g/1 -> Divide/2, cal gb/2(g)
  a/1 -> Sum2/1
  Sum2/1 -> Divide/1
  cal gb/1(gb) -> Sum2/2, gb/1
  DCM/1 -> cal gb/1(DCM)

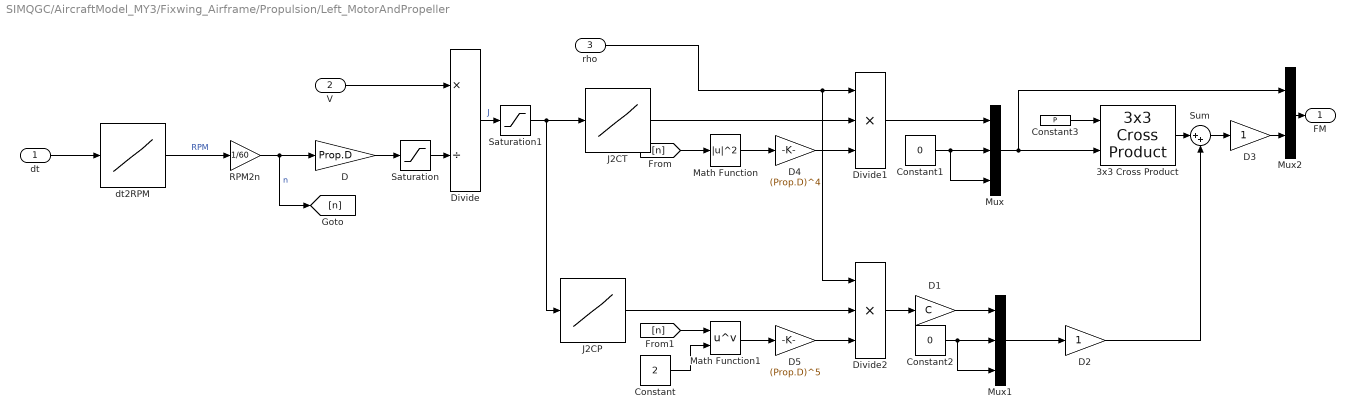
== system SIMQGC/AircraftModel_MY3/Fixwing_Airframe/Propulsion/Left_MotorAndPropeller ==
  dt : Inport
  V : Inport  Port=2
  rho : Inport  Port=3
  3x3 Cross Product : sharedutil/3x3 Cross Product
  Constant : Constant  Value=2
  Constant1 : Constant  Value=0
  Constant2 : Constant  Value=0
  Constant3 : Constant  Value=P
  D : Gain  Gain=Prop.D
  D1 : Gain  Gain=C
  D2 : Gain
  D3 : Gain
  D4 : Gain  Gain=(Prop.D)^4
  D5 : Gain  Gain=(Prop.D)^5
  Divide : Product  Inputs=*/
  Divide1 : Product  Inputs=***
  Divide2 : Product  Inputs=***
  J2CP : Lookup_n-D  NumberOfTableDimensions=1  BreakpointsForDimension1=Prop.J  Table=Prop.CP  InternalRulePriority=Speed  RndMeth=Simplest  InputSameDT=on
  J2CT : Lookup_n-D  NumberOfTableDimensions=1  BreakpointsForDimension1=Prop.J  Table=Prop.CT  InternalRulePriority=Speed  RndMeth=Simplest  InputSameDT=on
  Math Function : Math  Operator=magnitude^2  SaturateOnIntegerOverflow=on
  Math Function1 : Math  Operator=pow  SaturateOnIntegerOverflow=on
  Mux : Mux  Inputs=3
  Mux1 : Mux  Inputs=3
  Mux2 : Mux  Inputs=2
  RPM2n : Gain  Gain=1/60
  Saturation : Saturate  UpperLimit=inf  LowerLimit=1
  Saturation1 : Saturate  UpperLimit=0.79  LowerLimit=0  ZeroCross=off
  Sum : Sum  Inputs=|++
  dt2RPM : Lookup_n-D  NumberOfTableDimensions=1  BreakpointsForDimension1=Motor.dt  Table=Motor.rpm  InternalRulePriority=Speed  RndMeth=Simplest  InputSameDT=on
  FM : Outport
  wires:
  dt/1 -> dt2RPM/1
  dt2RPM/1 -> RPM2n/1  "RPM"
  RPM2n/1 -> [n], D/1  "n"
  D/1 -> Saturation/1
  V/1 -> Divide/1
  Divide/1 -> Saturation1/1  "J"
  rho/1 -> Divide2/1, Divide1/1
  J2CT/1 -> Divide1/2
  [n] -> Math Function/1
  Math Function/1 -> D4/1
  D4/1 -> Divide1/3
  J2CP/1 -> Divide2/2
  Math Function1/1 -> D5/1
  [n] -> Math Function1/1
  D5/1 -> Divide2/3
  Constant/1 -> Math Function1/2
  Divide1/1 -> Mux/1
  Constant1/1 -> Mux/3, Mux/2
  Divide2/1 -> D1/1
  D1/1 -> Mux1/1
  Constant2/1 -> Mux1/3, Mux1/2
  Mux/1 -> Mux2/1, 3x3 Cross Product/2
  Constant3/1 -> 3x3 Cross Product/1
  3x3 Cross Product/1 -> Sum/1
  Mux2/1 -> FM/1
  Saturation/1 -> Divide/2
  Saturation1/1 -> J2CT/1, J2CP/1
  Mux1/1 -> D2/1
  D2/1 -> Sum/2
  Sum/1 -> D3/1
  D3/1 -> Mux2/2

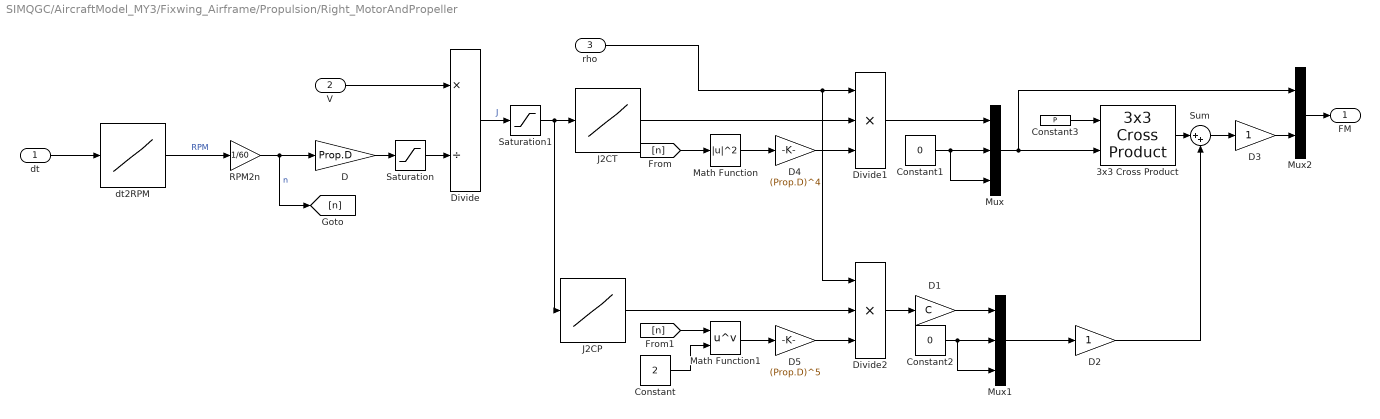
== system SIMQGC/AircraftModel_MY3/Fixwing_Airframe/Propulsion/Right_MotorAndPropeller ==
  dt : Inport
  V : Inport  Port=2
  rho : Inport  Port=3
  3x3 Cross Product : sharedutil/3x3 Cross Product
  Constant : Constant  Value=2
  Constant1 : Constant  Value=0
  Constant2 : Constant  Value=0
  Constant3 : Constant  Value=P
  D : Gain  Gain=Prop.D
  D1 : Gain  Gain=C
  D2 : Gain
  D3 : Gain
  D4 : Gain  Gain=(Prop.D)^4
  D5 : Gain  Gain=(Prop.D)^5
  Divide : Product  Inputs=*/
  Divide1 : Product  Inputs=***
  Divide2 : Product  Inputs=***
  J2CP : Lookup_n-D  NumberOfTableDimensions=1  BreakpointsForDimension1=Prop.J  Table=Prop.CP  InternalRulePriority=Speed  RndMeth=Simplest  InputSameDT=on
  J2CT : Lookup_n-D  NumberOfTableDimensions=1  BreakpointsForDimension1=Prop.J  Table=Prop.CT  InternalRulePriority=Speed  RndMeth=Simplest  InputSameDT=on
  Math Function : Math  Operator=magnitude^2  SaturateOnIntegerOverflow=on
  Math Function1 : Math  Operator=pow  SaturateOnIntegerOverflow=on
  Mux : Mux  Inputs=3
  Mux1 : Mux  Inputs=3
  Mux2 : Mux  Inputs=2
  RPM2n : Gain  Gain=1/60
  Saturation : Saturate  UpperLimit=inf  LowerLimit=1
  Saturation1 : Saturate  UpperLimit=0.79  LowerLimit=0  ZeroCross=off
  Sum : Sum  Inputs=|++
  dt2RPM : Lookup_n-D  NumberOfTableDimensions=1  BreakpointsForDimension1=Motor.dt  Table=Motor.rpm  InternalRulePriority=Speed  RndMeth=Simplest  InputSameDT=on
  FM : Outport
  wires:
  Mux2/1 -> FM/1
  Sum/1 -> D3/1
  3x3 Cross Product/1 -> Sum/1
  Constant3/1 -> 3x3 Cross Product/1
  Mux/1 -> 3x3 Cross Product/2, Mux2/1
  Constant2/1 -> Mux1/2, Mux1/3
  D1/1 -> Mux1/1
  Divide2/1 -> D1/1
  Constant1/1 -> Mux/2, Mux/3
  Divide1/1 -> Mux/1
  Constant/1 -> Math Function1/2
  D5/1 -> Divide2/3
  [n] -> Math Function1/1
  Math Function1/1 -> D5/1
  J2CP/1 -> Divide2/2
  D4/1 -> Divide1/3
  Math Function/1 -> D4/1
  [n] -> Math Function/1
  J2CT/1 -> Divide1/2
  rho/1 -> Divide1/1, Divide2/1
  Divide/1 -> Saturation1/1  "J"
  V/1 -> Divide/1
  D/1 -> Saturation/1
  RPM2n/1 -> D/1, [n]  "n"
  dt2RPM/1 -> RPM2n/1  "RPM"
  dt/1 -> dt2RPM/1
  Saturation/1 -> Divide/2
  Saturation1/1 -> J2CT/1, J2CP/1
  Mux1/1 -> D2/1
  D2/1 -> Sum/2
  D3/1 -> Mux2/2

== system SIMQGC/AircraftModel_MY3/Fixwing_Airframe/Aerodynamics/Aerodynamic Coefficients/Basic Coefficients ==
  alpha : Inport
  beta : Inport  Port=2
  mach : Inport  Port=3
  Sum : Sum  Inputs=|++
  alat : Subsystem
  alon : Subsystem
  coeff : Outport
  wires:
  alpha/1 -> alon/1(alpha), alat/2(alpha)
  beta/1 -> alat/1(beta)
  mach/1 -> alon/2(Mach)
  alat/1(alat) -> Sum/1
  alon/1(alon) -> Sum/2
  Sum/1 -> coeff/1

== system SIMQGC/AircraftModel_MY3/Fixwing_Airframe/Aerodynamics/Aerodynamic Coefficients/Body Rate Damping ==
  alpha : Inport
  pqrn : Inport  Port=2
  Demux : Demux  Outputs=3
  Product : Product  SaturateOnIntegerOverflow=on  InputSameDT=on  OutDataTypeStr=Inherit: Same as first input
  Product1 : Product  SaturateOnIntegerOverflow=on  InputSameDT=on  OutDataTypeStr=Inherit: Same as first input
  Product2 : Product  SaturateOnIntegerOverflow=on  InputSameDT=on  OutDataTypeStr=Inherit: Same as first input
  Sum1 : Sum  Inputs=+++  SaturateOnIntegerOverflow=on  InputSameDT=on  OutDataTypeStr=Inherit: Same as first input
  adyn : Subsystem
  coeff : Outport
  wires:
  Sum1/1 -> coeff/1
  Product1/1 -> Sum1/2
  Product2/1 -> Sum1/3
  Product/1 -> Sum1/1
  pqrn/1 -> Demux/1
  Demux/1 -> Product/2
  Demux/2 -> Product1/2
  Demux/3 -> Product2/2
  alpha/1 -> adyn/1(alpha)
  adyn/1(pout) -> Product/1
  adyn/2(qout) -> Product1/1
  adyn/3(rout) -> Product2/1

== system SIMQGC/AircraftModel_MY3/Fixwing_Airframe/Aerodynamics/Aerodynamic Coefficients/actuator ==
  alpha : Inport
  act : Inport  Port=2
  Bus Selector6 : BusSelector  OutputSignals=de
  ade : Subsystem
  coeff : Outport
  wires:
  act/1 -> Bus Selector6/1
  Bus Selector6/1 -> ade/2(de)  "<de>"
  alpha/1 -> ade/1(alpha)
  ade/1(Coeff) -> coeff/1

== system SIMQGC/AircraftModel_MY3/Fixwing_Airframe/Aerodynamics/Aerodynamic Coefficients/body axis forces ==
  alpha : Inport
  beta : Inport  Port=2
  Cl_LDY : Inport  Port=3
  Cl_xA : Fcn  Expr=-u[4]*cos(u[2])*cos(u[1])+u[3]*sin(u[1])
  Cl_yA : Fcn  Expr=-u[4]*sin(u[2])+u[5]
  Cl_zA : Fcn  Expr=-u[4]*cos(u[2])*sin(u[1])-u[3]*cos(u[1])
  Mux : Mux  Inputs=3
  Mux1 : Mux  Inputs=3
  Cl_XYZ : Outport
  wires:
  beta/1 -> Mux1/2
  Cl_LDY/1 -> Mux1/3
  Mux1/1 -> Cl_xA/1, Cl_yA/1, Cl_zA/1
  Cl_xA/1 -> Mux/1
  Cl_yA/1 -> Mux/2
  Cl_zA/1 -> Mux/3
  alpha/1 -> Mux1/1
  Mux/1 -> Cl_XYZ/1

== system SIMQGC/AircraftModel_MY3/Fixwing_Airframe/Aerodynamics/DerivedConditions1/Incidence, Sideslip, & Airspeed ==
  Vb : Inport
  Airspeed : Sqrt  AlgorithmType=Newton-Raphson  SaturateOnIntegerOverflow=on
  Allow All : UnitConfiguration  UnitSystemsStr=English,SI,SI (extended)  AllowAllUnitSystems=off
  Incidence : Trigonometry  Operator=atan2
  Product : Product  Inputs=*/  SaturateOnIntegerOverflow=on  OutDataTypeStr=Inherit: Same as first input
  Saturation : Saturate  UpperLimit=inf  LowerLimit=0.1
  Sideslip : Trigonometry  Operator=asin
  Subsystem : Subsystem
  Subsystem1 : Subsystem
  dot : Subsystem
  Alpha : Outport  Unit=rad  InitialOutput=0
  Beta : Outport  Port=2  Unit=rad  InitialOutput=0
  V : Outport  Port=3  InitialOutput=0
  wires:
  Product/1 -> Sideslip/1
  Subsystem/1(w) -> Incidence/1
  Subsystem/2(U) -> Incidence/2
  dot/1(dot) -> Airspeed/1
  Airspeed/1 -> Saturation/1, V/1
  Incidence/1 -> Alpha/1
  Vb/1 -> Subsystem/1(V), Subsystem1/1(V), dot/1(Vb)
  Sideslip/1 -> Beta/1
  Subsystem1/1(v) -> Product/1
  Saturation/1 -> Product/2

== system SIMQGC/AircraftModel_MY3/Fixwing_Airframe/Aerodynamics/DerivedConditions1/gamma chi & speed ==
  Ve : Inport
  Demux1 : Demux  Outputs=3
  Gain : Gain  Gain=-1
  Incidence : Trigonometry  Operator=atan2
  Product : Product  Inputs=*/  SaturateOnIntegerOverflow=on  OutDataTypeStr=Inherit: Same as first input
  Saturation : Saturate  UpperLimit=inf  LowerLimit=0.1
  azimuth : Trigonometry  Operator=asin
  norm : Subsystem
  gamma : Outport
  chi : Outport  Port=2
  V : Outport  Port=3
  wires:
  Gain/1 -> Product/1
  Product/1 -> azimuth/1
  azimuth/1 -> gamma/1
  norm/1(n) -> Saturation/1
  Demux1/1 -> Incidence/2, norm/1(x)
  Demux1/2 -> Incidence/1, norm/2(y)
  Demux1/3 -> Gain/1, norm/3(z)
  Ve/1 -> Demux1/1
  Incidence/1 -> chi/1
  Saturation/1 -> V/1, Product/2

== system SIMQGC/AircraftModel_MY3/Fixwing_Airframe/GroundForces/LF_Gear/GenerateGroundFM1 ==
  zrw : Inport
  Xgb : Inport  Port=2
  DCM : Inport  Port=3
  ze : Inport  Port=4
  Vb : Inport  Port=5
  pqr : Inport  Port=6
  psi : Inport  Port=7
  Enable : EnablePort  PropagateVarSize=During execution
  Calc Gear Force and Pos : Subsystem
  Calc Tire Force : Subsystem
  Gear Local Force vector : Concatenate  Mode=Multidimensional array
  LocMatrix : Subsystem
  Local Forces to Body Axes : Product  Multiplication=Matrix(*)  SaturateOnIntegerOverflow=on  InputSameDT=on  OutDataTypeStr=Inherit: Same as first input
  Mux2 : Mux  Inputs=2
  Selector2 : Selector  InputPortWidth=3  IndexOptions=Index vector (dialog)  Indices=1  OutputSizes=1
  Selector3 : Selector  InputPortWidth=3  IndexOptions=Index vector (dialog)  Indices=2  OutputSizes=1
  Transpose1 : Math  Operator=transpose  SaturateOnIntegerOverflow=on
  force to moment : Product  Multiplication=Matrix(*)  SaturateOnIntegerOverflow=on  InputSameDT=on  OutDataTypeStr=Inherit: Same as first input
  S : Outport
  FM : Outport  Port=2
  wires:
  [Fz] -> Gear Local Force vector/2, Calc Tire Force/6(Fz)
  psi/1 -> Calc Tire Force/4(psi)
  pqr/1 -> Calc Tire Force/3(pqr)
  Vb/1 -> Calc Tire Force/2(Vb)
  Calc Tire Force/1(Fxyb) -> Gear Local Force vector/1
  Xgb/1 -> Selector2/1, Selector3/1, Calc Gear Force and Pos/1(Xgb)
  [LocMatrix] -> Calc Tire Force/5(LocMatrix)
  [LocMatrix] -> Transpose1/1
  LocMatrix/1(A) -> [LocMatrix]
  Mux2/1 -> FM/1
  force to moment/1 -> Mux2/2
  ze/1 -> Calc Gear Force and Pos/3(zcg)
  zrw/1 -> Calc Gear Force and Pos/2(zrw)
  DCM/1 -> Local Forces to Body Axes/1, Calc Tire Force/1(DCM), Calc Gear Force and Pos/4(DCM)
  Gear Local Force vector/1 -> Local Forces to Body Axes/2
  Selector3/1 -> LocMatrix/2(ygb)
  Selector2/1 -> LocMatrix/1(xgb)
  Transpose1/1 -> force to moment/1
  Local Forces to Body Axes/1 -> Mux2/1, force to moment/2
  Calc Gear Force and Pos/2(S_strut1) -> S/1
  Calc Gear Force and Pos/1(Fz1) -> [Fz]
  Calc Gear Force and Pos/3(zgb1) -> LocMatrix/3(zgb)
  Calc Tire Force/2(WgL) -> [WgL]
  [WgL] -> Calc Gear Force and Pos/5(WgL)

== system SIMQGC/AircraftModel_MY3/Fixwing_Airframe/GroundForces/LF_Gear/detect ground contact ==
  note: height of gear lowest point
  ze : Inport
  DCM : Inport  Port=2
  Xgb : Inport  Port=3
  Hrw : Inport  Port=4
  Gain2 : Gain  Gain=-1
  Rotate pos to body axes : Product  Multiplication=Matrix(*)  SaturateOnIntegerOverflow=on  InputSameDT=on  OutDataTypeStr=Inherit: Same as first input
  Sum2 : Sum  Inputs=|++
  Sum4 : Sum  Inputs=++|
  Transpose : Math  Operator=transpose  SaturateOnIntegerOverflow=on
  Zg : Selector  InputPortWidth=3  IndexOptions=Index vector (dialog)  Indices=3  OutputSizes=1
  detect_WOW : RelationalOperator  Operator=<=  OutDataTypeStr=boolean  RndMeth=Nearest
  radius of wheel : Constant  Value=Rw  VectorParams1D=off
  WOW : Outport
  wires:
  detect_WOW/1 -> WOW/1
  ze/1 -> Sum4/1
  Hrw/1 -> detect_WOW/2
  Xgb/1 -> Rotate pos to body axes/2
  DCM/1 -> Transpose/1
  Rotate pos to body axes/1 -> Zg/1
  Sum4/1 -> Sum2/1
  Sum2/1 -> Gain2/1
  Gain2/1 -> detect_WOW/1
  Zg/1 -> Sum4/2
  Transpose/1 -> Rotate pos to body axes/1
  radius of wheel/1 -> Sum2/2

== system SIMQGC/AircraftModel_MY3/Fixwing_Airframe/GroundForces/LM_Gear/GenerateGroundFM1 ==
  zrw : Inport
  Xgb : Inport  Port=2
  DCM : Inport  Port=3
  ze : Inport  Port=4
  Vb : Inport  Port=5
  pqr : Inport  Port=6
  psi : Inport  Port=7
  Enable : EnablePort  PropagateVarSize=During execution
  Calc Gear Force and Pos : Subsystem
  Calc Tire Force : Subsystem
  Gear Local Force vector : Concatenate  Mode=Multidimensional array
  LocMatrix : Subsystem
  Local Forces to Body Axes : Product  Multiplication=Matrix(*)  SaturateOnIntegerOverflow=on  InputSameDT=on  OutDataTypeStr=Inherit: Same as first input
  Mux2 : Mux  Inputs=2
  Selector2 : Selector  InputPortWidth=3  IndexOptions=Index vector (dialog)  Indices=1  OutputSizes=1
  Selector3 : Selector  InputPortWidth=3  IndexOptions=Index vector (dialog)  Indices=2  OutputSizes=1
  Transpose1 : Math  Operator=transpose  SaturateOnIntegerOverflow=on
  force to moment : Product  Multiplication=Matrix(*)  SaturateOnIntegerOverflow=on  InputSameDT=on  OutDataTypeStr=Inherit: Same as first input
  S : Outport
  FM : Outport  Port=2
  wires:
  [Fz] -> Gear Local Force vector/2, Calc Tire Force/6(Fz)
  psi/1 -> Calc Tire Force/4(psi)
  pqr/1 -> Calc Tire Force/3(pqr)
  Vb/1 -> Calc Tire Force/2(Vb)
  Calc Tire Force/1(Fxyb) -> Gear Local Force vector/1
  Xgb/1 -> Selector2/1, Selector3/1, Calc Gear Force and Pos/1(Xgb)
  [LocMatrix] -> Calc Tire Force/5(LocMatrix)
  [LocMatrix] -> Transpose1/1
  LocMatrix/1(A) -> [LocMatrix]
  Mux2/1 -> FM/1
  force to moment/1 -> Mux2/2
  ze/1 -> Calc Gear Force and Pos/3(zcg)
  zrw/1 -> Calc Gear Force and Pos/2(zrg)
  DCM/1 -> Local Forces to Body Axes/1, Calc Tire Force/1(DCM), Calc Gear Force and Pos/4(DCM)
  Gear Local Force vector/1 -> Local Forces to Body Axes/2
  Selector3/1 -> LocMatrix/2(ygb)
  Selector2/1 -> LocMatrix/1(xgb)
  Transpose1/1 -> force to moment/1
  Local Forces to Body Axes/1 -> Mux2/1, force to moment/2
  Calc Gear Force and Pos/2(S_strut1) -> S/1
  Calc Gear Force and Pos/1(Fz1) -> [Fz]
  Calc Gear Force and Pos/3(zgb1) -> LocMatrix/3(zgb)
  Calc Tire Force/2(WgL) -> [WgL]
  [WgL] -> Calc Gear Force and Pos/5(WgL)

== system SIMQGC/AircraftModel_MY3/Fixwing_Airframe/GroundForces/LM_Gear/detect ground contact ==
  note: height of gear lowest point
  ze : Inport
  DCM : Inport  Port=2
  Xgb : Inport  Port=3
  Hrw : Inport  Port=4
  Gain2 : Gain  Gain=-1
  Rotate pos to body axes : Product  Multiplication=Matrix(*)  SaturateOnIntegerOverflow=on  InputSameDT=on  OutDataTypeStr=Inherit: Same as first input
  Sum2 : Sum  Inputs=|++
  Sum4 : Sum  Inputs=++|
  Transpose : Math  Operator=transpose  SaturateOnIntegerOverflow=on
  Zg : Selector  InputPortWidth=3  IndexOptions=Index vector (dialog)  Indices=3  OutputSizes=1
  detect_WOW : RelationalOperator  Operator=<=  OutDataTypeStr=boolean  RndMeth=Nearest
  radius of wheel : Constant  Value=Rw  VectorParams1D=off
  WOW : Outport
  wires:
  detect_WOW/1 -> WOW/1
  ze/1 -> Sum4/1
  Hrw/1 -> detect_WOW/2
  Xgb/1 -> Rotate pos to body axes/2
  DCM/1 -> Transpose/1
  Rotate pos to body axes/1 -> Zg/1
  Sum4/1 -> Sum2/1
  Sum2/1 -> Gain2/1
  Gain2/1 -> detect_WOW/1
  Zg/1 -> Sum4/2
  Transpose/1 -> Rotate pos to body axes/1
  radius of wheel/1 -> Sum2/2

== system SIMQGC/AircraftModel_MY3/Fixwing_Airframe/GroundForces/LN_Gear/GenerateGroundFM1 ==
  zrw : Inport
  Xgb : Inport  Port=2
  DCM : Inport  Port=3
  ze : Inport  Port=4
  Vb : Inport  Port=5
  pqr : Inport  Port=6
  psi : Inport  Port=7
  Enable : EnablePort  PropagateVarSize=During execution
  Calc Gear Force and Pos : Subsystem
  Calc Tire Force : Subsystem
  Gear Local Force vector : Concatenate  Mode=Multidimensional array
  LocMatrix : Subsystem
  Local Forces to Body Axes : Product  Multiplication=Matrix(*)  SaturateOnIntegerOverflow=on  InputSameDT=on  OutDataTypeStr=Inherit: Same as first input
  Mux2 : Mux  Inputs=2
  Selector2 : Selector  InputPortWidth=3  IndexOptions=Index vector (dialog)  Indices=1  OutputSizes=1
  Selector3 : Selector  InputPortWidth=3  IndexOptions=Index vector (dialog)  Indices=2  OutputSizes=1
  Transpose1 : Math  Operator=transpose  SaturateOnIntegerOverflow=on
  force to moment : Product  Multiplication=Matrix(*)  SaturateOnIntegerOverflow=on  InputSameDT=on  OutDataTypeStr=Inherit: Same as first input
  S : Outport
  FM : Outport  Port=2
  wires:
  [Fz] -> Gear Local Force vector/2, Calc Tire Force/6(Fz)
  psi/1 -> Calc Tire Force/4(psi)
  pqr/1 -> Calc Tire Force/3(pqr)
  Vb/1 -> Calc Tire Force/2(Vb)
  Calc Tire Force/1(Fxyb) -> Gear Local Force vector/1
  Xgb/1 -> Selector2/1, Selector3/1, Calc Gear Force and Pos/1(Xgb)
  [LocMatrix] -> Calc Tire Force/5(LocMatrix)
  [LocMatrix] -> Transpose1/1
  LocMatrix/1(A) -> [LocMatrix]
  Mux2/1 -> FM/1
  force to moment/1 -> Mux2/2
  ze/1 -> Calc Gear Force and Pos/3(zcg)
  zrw/1 -> Calc Gear Force and Pos/2(zrg)
  DCM/1 -> Local Forces to Body Axes/1, Calc Tire Force/1(DCM), Calc Gear Force and Pos/4(DCM)
  Gear Local Force vector/1 -> Local Forces to Body Axes/2
  Selector3/1 -> LocMatrix/2(ygb)
  Selector2/1 -> LocMatrix/1(xgb)
  Transpose1/1 -> force to moment/1
  Local Forces to Body Axes/1 -> Mux2/1, force to moment/2
  Calc Gear Force and Pos/2(S_strut1) -> S/1
  Calc Gear Force and Pos/1(Fz1) -> [Fz]
  Calc Gear Force and Pos/3(zgb1) -> LocMatrix/3(zgb)
  Calc Tire Force/2(WgL) -> [WgL]
  [WgL] -> Calc Gear Force and Pos/5(WgL)

== system SIMQGC/AircraftModel_MY3/Fixwing_Airframe/GroundForces/LN_Gear/detect ground contact ==
  note: height of gear lowest point
  ze : Inport
  DCM : Inport  Port=2
  Xgb : Inport  Port=3
  Hrw : Inport  Port=4
  Gain2 : Gain  Gain=-1
  Rotate pos to body axes : Product  Multiplication=Matrix(*)  SaturateOnIntegerOverflow=on  InputSameDT=on  OutDataTypeStr=Inherit: Same as first input
  Sum2 : Sum  Inputs=|++
  Sum4 : Sum  Inputs=++|
  Transpose : Math  Operator=transpose  SaturateOnIntegerOverflow=on
  Zg : Selector  InputPortWidth=3  IndexOptions=Index vector (dialog)  Indices=3  OutputSizes=1
  detect_WOW : RelationalOperator  Operator=<=  OutDataTypeStr=boolean  RndMeth=Nearest
  radius of wheel : Constant  Value=Rw  VectorParams1D=off
  WOW : Outport
  wires:
  radius of wheel/1 -> Sum2/2
  Transpose/1 -> Rotate pos to body axes/1
  Zg/1 -> Sum4/2
  Gain2/1 -> detect_WOW/1
  Sum2/1 -> Gain2/1
  Sum4/1 -> Sum2/1
  Rotate pos to body axes/1 -> Zg/1
  DCM/1 -> Transpose/1
  Xgb/1 -> Rotate pos to body axes/2
  Hrw/1 -> detect_WOW/2
  ze/1 -> Sum4/1
  detect_WOW/1 -> WOW/1

== system SIMQGC/AircraftModel_MY3/Fixwing_Airframe/GroundForces/RF_Gear/GenerateGroundFM1 ==
  zrw : Inport
  Xgb : Inport  Port=2
  DCM : Inport  Port=3
  ze : Inport  Port=4
  Vb : Inport  Port=5
  pqr : Inport  Port=6
  psi : Inport  Port=7
  Enable : EnablePort  PropagateVarSize=During execution
  Calc Gear Force and Pos : Subsystem
  Calc Tire Force : Subsystem
  Gear Local Force vector : Concatenate  Mode=Multidimensional array
  LocMatrix : Subsystem
  Local Forces to Body Axes : Product  Multiplication=Matrix(*)  SaturateOnIntegerOverflow=on  InputSameDT=on  OutDataTypeStr=Inherit: Same as first input
  Mux2 : Mux  Inputs=2
  Selector2 : Selector  InputPortWidth=3  IndexOptions=Index vector (dialog)  Indices=1  OutputSizes=1
  Selector3 : Selector  InputPortWidth=3  IndexOptions=Index vector (dialog)  Indices=2  OutputSizes=1
  Transpose1 : Math  Operator=transpose  SaturateOnIntegerOverflow=on
  force to moment : Product  Multiplication=Matrix(*)  SaturateOnIntegerOverflow=on  InputSameDT=on  OutDataTypeStr=Inherit: Same as first input
  S : Outport
  FM : Outport  Port=2
  wires:
  [Fz] -> Gear Local Force vector/2, Calc Tire Force/6(Fz)
  psi/1 -> Calc Tire Force/4(psi)
  pqr/1 -> Calc Tire Force/3(pqr)
  Vb/1 -> Calc Tire Force/2(Vb)
  Calc Tire Force/1(Fxyb) -> Gear Local Force vector/1
  Xgb/1 -> Selector2/1, Selector3/1, Calc Gear Force and Pos/1(Xgb)
  [LocMatrix] -> Calc Tire Force/5(LocMatrix)
  [LocMatrix] -> Transpose1/1
  LocMatrix/1(A) -> [LocMatrix]
  Mux2/1 -> FM/1
  force to moment/1 -> Mux2/2
  ze/1 -> Calc Gear Force and Pos/3(zcg)
  zrw/1 -> Calc Gear Force and Pos/2(zrg)
  DCM/1 -> Local Forces to Body Axes/1, Calc Tire Force/1(DCM), Calc Gear Force and Pos/4(DCM)
  Gear Local Force vector/1 -> Local Forces to Body Axes/2
  Selector3/1 -> LocMatrix/2(ygb)
  Selector2/1 -> LocMatrix/1(xgb)
  Transpose1/1 -> force to moment/1
  Local Forces to Body Axes/1 -> Mux2/1, force to moment/2
  Calc Gear Force and Pos/2(S_strut1) -> S/1
  Calc Gear Force and Pos/1(Fz1) -> [Fz]
  Calc Gear Force and Pos/3(zgb1) -> LocMatrix/3(zgb)
  Calc Tire Force/2(WgL) -> [WgL]
  [WgL] -> Calc Gear Force and Pos/5(WgL)
